simulink model "Question_7_SL"  (R2017a)
settings: Solver=VariableStepAuto  StartTime=0.0  StopTime=10.0  RelTol=1e-3
libraries: simulink x2
settings Model: Creator=rashaf01  LastModifiedBy=vonl01

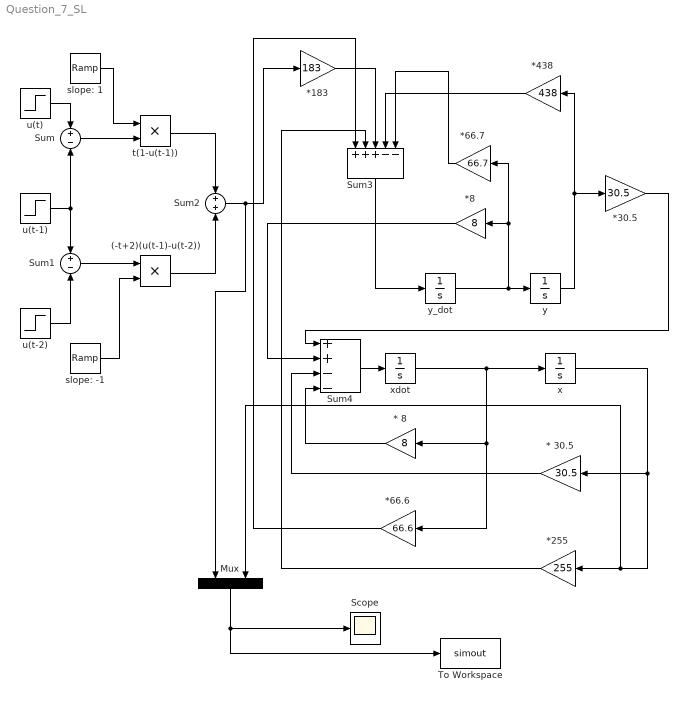
== system Question_7_SL ==
  (-t+2)(u(t-1)-u(t-2)) : Product
  * 30.5 : Gain  Gain=30.5
  * 8 : Gain  Gain=8
  *183 : Gain  Gain=183
  "*255 " : Gain  Gain=255
  *30.5 : Gain  Gain=30.5
  *438 : Gain  Gain=438
  *66.6 : Gain  Gain=66.6
  *66.7 : Gain  Gain=66.7
  *8 : Gain  Gain=8
  Mux : Mux  Inputs=2
  Scope : Scope
  Sum : Sum  Inputs=+-
  Sum1 : Sum  Inputs=+-
  Sum2 : Sum
  Sum3 : Sum  Inputs=+++--
  Sum4 : Sum  Inputs=++--
  To Workspace : ToWorkspace  VariableName=simout  SampleTime=-1
  slope: -1 : simulink/Sources/Ramp  slope=-1  start=0  X0=2
  slope: 1 : simulink/Sources/Ramp  slope=1  start=0  X0=0
  t(1-u(t-1)) : Product
  u(t) : Step  Time=0  SampleTime=0
  u(t-1) : Step  SampleTime=0
  u(t-2) : Step  Time=2  SampleTime=0
  x : Integrator
  xdot : Integrator
  y : Integrator
  y_dot : Integrator
  wires:
  u(t)/1 -> Sum/1
  u(t-1)/1 -> Sum/2, Sum1/1
  Sum/1 -> t(1-u(t-1))/2
  slope: 1/1 -> t(1-u(t-1))/1
  t(1-u(t-1))/1 -> Sum2/1
  (-t+2)(u(t-1)-u(t-2))/1 -> Sum2/2
  u(t-2)/1 -> Sum1/2
  Sum1/1 -> (-t+2)(u(t-1)-u(t-2))/1
  slope: -1/1 -> (-t+2)(u(t-1)-u(t-2))/2
  Sum2/1 -> Mux/1, *183/1
  *183/1 -> Sum3/3
  *438/1 -> Sum3/4
  *66.7/1 -> Sum3/5
  Sum3/1 -> y_dot/1
  *8/1 -> Sum4/2
  y_dot/1 -> *66.7/1, *8/1, y/1
  y/1 -> *30.5/1, *438/1
  *30.5/1 -> Sum4/1
  Sum4/1 -> xdot/1
  xdot/1 -> *66.6/1, * 8/1, x/1
  * 8/1 -> Sum4/4
  x/1 -> "*255 "/1, Mux/2, * 30.5/1
  * 30.5/1 -> Sum4/3
  *66.6/1 -> Sum3/1
  "*255 "/1 -> Sum3/2
  Mux/1 -> To Workspace/1, Scope/1
